simulink model "eCS_Algo_Simulation_2015b_opti - original"  (R2015b)
settings: Solver=ode1  StartTime=0.0  StopTime=3  FixedStep=1/80000  RelTol=1e-3
PreLoadFcn:
  | if exist('tl_preloadfcn','file'), tl_preloadfcn(gcs,402); end
PostLoadFcn:
  | , if any(exist('dsrtsu_mdlpostloadfcn', 'file') == [2, 3, 6]), try dsrtsu_mdlpostloadfcn('Execute', bdroot); catch fprintf('Error in PostLoadFcn (dsrtsu_mdlpostloadfcn) for model "%s":\n %s\n', bdroot, lasterr); end, end,
  | if exist('tl_postloadfcn','file'), tl_postloadfcn(gcs,402); end
InitFcn:
  | Omegan=1.3024e+03;
  | xi=0.9; %0.48
  | K=0.1931;
  | K1=0.0198;
  | TauLocked=0.00255;
  | TauUnLocked=0.0042;
  | Kp=1/(2*K1);
  | Ki=Kp/((TauLocked+TauUnLocked)/2);
  | if exist('tlds_init','file'), tlds_init(gcs); end
StartFcn:
  | if exist('tlds_start','file'), tlds_start(gcs); end
StopFcn:
  | if exist('tlds_stop','file'), tlds_stop(gcs); end
model workspace (MAT data in the model file):
  au8PrevExecProfile = [0 0 0 0 0 0]
values from neighbouring files (symbols this model uses):
  AccSensor = 5    [Parameter_eCS_Algo.m]
  AlgoType = 0    [Parameter_eCS_Algo.m]
  Cxy = 1*0.017    (= 0.017)    [Acc_Init_SelV1.m]
  Cxz = 1*0.017    (= 0.017)    [Acc_Init_SelV1.m]
  Cyx = 1*0.017    (= 0.017)    [Acc_Init_SelV1.m]
  Cyz = 1*0.017    (= 0.017)    [Acc_Init_SelV1.m]
  Czx = 1*0.017    (= 0.017)    [Acc_Init_SelV1.m]
  Czy = 1*0.017    (= 0.017)    [Acc_Init_SelV1.m]
  Forced_Oscillation = 0    [Parameter_eCS_Algo.m]    (also in run_Rotation_sim.m = run)
  FreqTemperature = 10    [Acc_Init_SelV1.m]
  MaxSensorOffset = 0.3    [Acc_Init_SelV1.m]
  Mean_x_noise = 4e-3    (= 0.004)    [Acc_Init_SelV1.m]
  Mean_y_noise = 4e-3    (= 0.004)    [Acc_Init_SelV1.m]
  Mean_z_noise = 4e-3    (= 0.004)    [Acc_Init_SelV1.m]
  ODR = 8000    [Acc_Init_SelV1.m]
  offsetcorrection_on_off = 0    [Parameter_eCS_Algo.m]
  phi_pulse_rotation = 0    [Parameter_eCS_Algo.m]    (also in run_Rotation_sim.m = angle)
  pulsetype = 2    [Parameter_eCS_Algo.m]    (also in run_simulation.m = j; run_simulation_ActiveX.m = j)
  Range = 4    [Acc_Init_SelV1.m]
  sensitivity_optimisation = 0    [Parameter_eCS_Algo.m]
  TempBias = 0    [Acc_Init_SelV1.m]
  TemperatureAmp = 0    [Acc_Init_SelV1.m]
  Var_x_noise = 1.84e-9    (= 1.84e-09)    [Acc_Init_SelV1.m]
  Var_y_noise = 2.025e-09    [Acc_Init_SelV1.m]
  Var_z_noise = 1.374e-09    [Acc_Init_SelV1.m]
  w_x = 2*pi*F_x    (= 376.991118431)    [Acc_Init_SelV1.m]
  w_y = 2*pi*F_y    (= 376.991118431)    [Acc_Init_SelV1.m]
  w_z = 2*pi*F_z    (= 376.991118431)    [Acc_Init_SelV1.m]
  x_max_temp_drift = 0.061    [Acc_Init_SelV1.m]
  x_offset_enable = 0    [Acc_Init_SelV1.m]
  x_run_to_run_drift = 0.0    (= 0)    [Acc_Init_SelV1.m]
  x_temp_co_drift = 0.000    (= 0)    [Acc_Init_SelV1.m]
  Xi_x = 0.7    [Acc_Init_SelV1.m]
  Xi_y = 0.7    [Acc_Init_SelV1.m]
  Xi_z = 0.7    [Acc_Init_SelV1.m]
  y_max_temp_drift = 0.061    [Acc_Init_SelV1.m]
  y_offset_enable = 0    [Acc_Init_SelV1.m]
  y_run_to_run_drift = 0.0    (= 0)    [Acc_Init_SelV1.m]
  y_temp_co_drift = 0.000    (= 0)    [Acc_Init_SelV1.m]
  z_max_temp_drift = 0.13    [Acc_Init_SelV1.m]
  z_offset_enable = 0    [Acc_Init_SelV1.m]
  z_run_to_run_drift = 0.0    (= 0)    [Acc_Init_SelV1.m]
  z_temp_co_drift = 0.000    (= 0)    [Acc_Init_SelV1.m]
undefined symbols (not defined in the file or in its folder): ddv, DiscIntNeverNeededParam, gmw_roada_x__m_s__, gmw_roada_y__m_s__, gmw_roadtime_2kHz, KSF_50_a_x, KSF_50_a_y, KSF_50_time, KSG_30_a_x, KSG_30_a_y, KSG_30_time, Meldorf_HindenburgstraAcceleration_x__m_s_2_, Meldorf_HindenburgstraAcceleration_y__m_s_2_, Meldorf_HindenburgstraAcceleration_z__m_s_2_, Meldorf_HindenburgstraTime__s_, pulse_FF27, pulse_MPDB, pulse_ODB40, pulse_ODB64, pulse_USNCAP, pulsetime_FF27, pulsetime_MPDB, pulsetime_ODB40, pulsetime_ODB64, pulsetime_USNCAP, Rauasphalt_60_a_x, Rauasphalt_60_a_y, Rauasphalt_60_time, sigbuilder_block, VW_416_2kHza_x_2kHz, VW_416_2kHza_y_2kHz, VW_416_2kHztime_2kHz
libraries: simulink x20, tllib x16, tl_autosar_lib x12, simulink_extras x7, LIB_TF_G_12_StepControl x2, LIB_TF_G_111 x1, LIB_TF_G_112 x1
(part 9 of 9)

== system eCS_Algo_Simulation_2015b_opti - original/SAD/Subsystem/SAD/SAD/SAD_runMainFunction/SAD mainfunction/ComputeDutyCycle/UnlockRequest/scp_GetCurrent ==
  u8TypeOfMeasure : Inport  PortDimensions=1  mask(TL_Inport){data={'autosar',{'useautosarcommunication',1,'kind',5,'operationargument','AUTOLIV/AdcIf_DataDictionnary/ClientServerInterfaces/icsConvertedAdcService/Operations/getMeasure/OperationArguments/u8TypeOfMeasure'},'date',738771.48216400458}}
      settings: CopyFcn=if exist('tl_reset_reviewflag') == 2, tl_reset_reviewflag(gcbh); end  DeleteFcn=if exist('delete_tlblock','file')==2,delete_tlblock(gcbh);end  NameChangeFcn=if exist('rename_tlblock','file')==2,rename_tlblock(gcbh);end  OpenFcn=if exist('tl_open_blockdlg','file')==2,tl_open_blockdlg(gcbh);else,open_system(gcbh,'parameter');end
      mask Help: eval(['if exist(''tl_online_help'',''file'') == 2, tl_online_help(''Topic'',''TL_Inport''),else, web([''jar:file:///'',matlabroot,''/help/toolbox/simulink/help.jar!/slref/' lower(get_param(gcbh,'Blocktype')) '.html''], ''-helpbrowser''),end'])
      mask Display: plot([0.2 0.35 NaN 0.65 0.8],[0 1 NaN 0 1]);
  Data Store Read : DataStoreRead  mask(TL_DataStoreRead){data={'date',738672.58044925926}}
      settings: DeleteFcn=if exist('delete_tlblock','file')==2,delete_tlblock(gcbh);end  NameChangeFcn=if exist('rename_tlblock','file')==2,rename_tlblock(gcbh);end  OpenFcn=if exist('tl_open_blockdlg','file')==2,tl_open_blockdlg(gcbh);else,open_system(gcbh,'parameter');end
      mask Help: eval(['if exist(''tl_online_help'',''file'') == 2, tl_online_help(''Topic'',''TL_DataStoreRead''),else, web([''jar:file:///'',matlabroot,''/help/toolbox/simulink/help.jar!/slref/' lower(get_param(gcbh,'Blocktype')) '.html''], ''-helpbrowser''),end'])
      mask Display: plot([-0.1, 1.05, NaN, -0.1, 1.05],[.01, .01, NaN, .99, .99]);
  Selector : Selector  IndexMode=Zero-based  InputPortWidth=6  IndexOptions=Index vector (port)  Indices=[1 3]  OutputSizes=1
  ServerCallPoint : tllib/Function  data={'autosar',{'useautosarspecification',1,'functionrole',3,'clientport','pclSolenoidCurrent','operation','getMeasure','clientsoftwarecomponent','AUTOLIV/SoftwareComponents/SAD/SAD'},'date',738770.65144107642}  displayString=|
      | OPERATION CALL
      | (SYNCHRONOUS)
  u16Current : Outport  PortDimensions=1  mask(TL_Outport){data={'autosar',{'useautosarcommunication',1,'kind',5,'operationargument','AUTOLIV/AdcIf_DataDictionnary/ClientServerInterfaces/icsConvertedAdcService/Operations/getMeasure/OperationArguments/u16Measure'},'date',738771.47910792823}}
      settings: CopyFcn=if exist('tl_reset_reviewflag') == 2, tl_reset_reviewflag(gcbh); end  DeleteFcn=if exist('delete_tlblock','file')==2,delete_tlblock(gcbh);end  NameChangeFcn=if exist('rename_tlblock','file')==2,rename_tlblock(gcbh);end  OpenFcn=if exist('tl_open_blockdlg','file')==2,tl_open_blockdlg(gcbh);else,open_system(gcbh,'parameter');end
      mask Help: eval(['if exist(''tl_online_help'',''file'') == 2, tl_online_help(''Topic'',''TL_Outport''),else, web([''jar:file:///'',matlabroot,''/help/toolbox/simulink/help.jar!/slref/' lower(get_param(gcbh,'Blocktype')) '.html''], ''-helpbrowser''),end'])
      mask Display: plot([0.2 0.35 NaN 0.65 0.8],[0 1 NaN 0 1]);
  wires:
  Selector/1 -> u16Current/1
  Data Store Read/1 -> Selector/1
  u8TypeOfMeasure/1 -> Selector/2

== system eCS_Algo_Simulation_2015b_opti - original/eCS/Subsystem/eCS/eCS/eCS_runMainFunction/Crash Acceleration/Acceleration Clipping/If Action Subsystem/Clear Trigger  ==
  u16OldTimer : Inport
  Action Port : ActionPort  ActionType=then
  Constant1 : Constant  Value=0  mask(TL_Constant){data={'date',738573.7192003472}}
      settings: CopyFcn=if exist('tl_reset_reviewflag') == 2, tl_reset_reviewflag(gcbh); end  DeleteFcn=if exist('delete_tlblock','file')==2,delete_tlblock(gcbh);end  NameChangeFcn=if exist('rename_tlblock','file')==2,rename_tlblock(gcbh);end  OpenFcn=if exist('tl_open_blockdlg','file')==2,tl_open_blockdlg(gcbh);else,open_system(gcbh,'parameter');end
      mask Help: eval(['if exist(''tl_online_help'',''file'') == 2, tl_online_help(''Topic'',''TL_Constant''),else, web([''jar:file:///'',matlabroot,''/help/toolbox/simulink/help.jar!/slref/' lower(get_param(gcbh,'Blocktype')) '.html''], ''-helpbrowser''),end'])
      mask Display: plot([-0.1, 1.05, NaN, -0.1, 1.05],[.01, .01, NaN, .99, .99]);
  Trigger : Outport  InitialOutput=0
  u16Timer : Outport  Port=2  InitialOutput=0
  wires:
  Constant1/1 -> Trigger/1
  u16OldTimer/1 -> u16Timer/1

== system eCS_Algo_Simulation_2015b_opti - original/eCS/Subsystem/eCS/eCS/eCS_runMainFunction/Crash Acceleration/Acceleration Clipping/If Action Subsystem/Decrease Timer ==
  u16OldTimer : Inport
  u8OldTrigger : Inport  Port=2
  Action Port : ActionPort  ActionType=else
  Constant : Constant  mask(TL_Constant){data={'date',738573.71920056711}}
      settings: CopyFcn=if exist('tl_reset_reviewflag') == 2, tl_reset_reviewflag(gcbh); end  DeleteFcn=if exist('delete_tlblock','file')==2,delete_tlblock(gcbh);end  NameChangeFcn=if exist('rename_tlblock','file')==2,rename_tlblock(gcbh);end  OpenFcn=if exist('tl_open_blockdlg','file')==2,tl_open_blockdlg(gcbh);else,open_system(gcbh,'parameter');end
      mask Help: eval(['if exist(''tl_online_help'',''file'') == 2, tl_online_help(''Topic'',''TL_Constant''),else, web([''jar:file:///'',matlabroot,''/help/toolbox/simulink/help.jar!/slref/' lower(get_param(gcbh,'Blocktype')) '.html''], ''-helpbrowser''),end'])
      mask Display: plot([-0.1, 1.05, NaN, -0.1, 1.05],[.01, .01, NaN, .99, .99]);
  Constant1 : Constant  Value=0  mask(TL_Constant){data={'date',738573.71920068283}}
      settings: CopyFcn=if exist('tl_reset_reviewflag') == 2, tl_reset_reviewflag(gcbh); end  DeleteFcn=if exist('delete_tlblock','file')==2,delete_tlblock(gcbh);end  NameChangeFcn=if exist('rename_tlblock','file')==2,rename_tlblock(gcbh);end  OpenFcn=if exist('tl_open_blockdlg','file')==2,tl_open_blockdlg(gcbh);else,open_system(gcbh,'parameter');end
      mask Help: eval(['if exist(''tl_online_help'',''file'') == 2, tl_online_help(''Topic'',''TL_Constant''),else, web([''jar:file:///'',matlabroot,''/help/toolbox/simulink/help.jar!/slref/' lower(get_param(gcbh,'Blocktype')) '.html''], ''-helpbrowser''),end'])
      mask Display: plot([-0.1, 1.05, NaN, -0.1, 1.05],[.01, .01, NaN, .99, .99]);
  HoldingTimer : Switch  Criteria=u2 ~= 0  mask(TL_Switch){data={'output',{'type','UInt16'},'date',738573.71920091438}}
      settings: CopyFcn=if exist('tl_reset_reviewflag') == 2, tl_reset_reviewflag(gcbh); end  DeleteFcn=if exist('delete_tlblock','file')==2,delete_tlblock(gcbh);end  NameChangeFcn=if exist('rename_tlblock','file')==2,rename_tlblock(gcbh);end  OpenFcn=if exist('tl_open_blockdlg','file')==2,tl_open_blockdlg(gcbh);else,open_system(gcbh,'parameter');end
      mask Help: eval(['if exist(''tl_online_help'',''file'') == 2, tl_online_help(''Topic'',''TL_Switch''),else, web([''jar:file:///'',matlabroot,''/help/toolbox/simulink/help.jar!/slref/' lower(get_param(gcbh,'Blocktype')) '.html''], ''-helpbrowser''),end'])
      mask Display: plot([-0.1, 1.05, NaN, -0.1, 1.05],[.01, .01, NaN, .99, .99]);
  Sum : Sum  Inputs=+-  mask(TL_Sum){data={'output',{'type','UInt16'},'date',738573.71920103009}}
      settings: CopyFcn=if exist('tl_reset_reviewflag') == 2, tl_reset_reviewflag(gcbh); end  DeleteFcn=if exist('delete_tlblock','file')==2,delete_tlblock(gcbh);end  NameChangeFcn=if exist('rename_tlblock','file')==2,rename_tlblock(gcbh);end  OpenFcn=if exist('tl_open_blockdlg','file')==2,tl_open_blockdlg(gcbh);else,open_system(gcbh,'parameter');end
      mask Help: eval(['if exist(''tl_online_help'',''file'') == 2, tl_online_help(''Topic'',''TL_Sum''),else, web([''jar:file:///'',matlabroot,''/help/toolbox/simulink/help.jar!/slref/' lower(get_param(gcbh,'Blocktype')) '.html''], ''-helpbrowser''),end'])
      mask Display: plot([-0.1, 1.05, NaN, -0.1, 1.05],[.01, .01, NaN, .99, .99]);
  u16Timer : Outport  InitialOutput=0
  Trigger : Outport  Port=2  InitialOutput=0
  wires:
  u16OldTimer/1 -> Sum/1, HoldingTimer/2
  HoldingTimer/1 -> u16Timer/1
  Constant/1 -> Sum/2
  Sum/1 -> HoldingTimer/1
  Constant1/1 -> HoldingTimer/3
  u8OldTrigger/1 -> Trigger/1

== matlab function eCS_Algo_Simulation_2015b_opti - original/retractor locking trigger ==
  settings: updateMethod=DISCRETE
  data: trigger_solenoid input; s input; s_mech_locking input; trigger_retractor output; time input; triggertime_retractor output; s_locking output
function [trigger_retractor,triggertime_retractor,s_locking]     = retractor_locking_trigger(trigger_solenoid, s, s_mech_locking,time)

%local variable declaration
persistent s_store
persistent trigger_old
persistent trigger_intern
persistent t_store
persistent s_locking_intern
persistent once

% Initialisation
if isempty(s_store)
    s_store=10000;
    trigger_old=0;
    trigger_intern=0;    
    t_store=0;
    s_locking_intern=0;
    once=0;
end


%main
if and(trigger_old==0, trigger_solenoid==1)
    trigger_old=1;
    s_store=s;
    %s_locking_intern=s;
end

if and(s-s_store>s_mech_locking , once==0)
    once=1;
    trigger_intern=1;
    t_store=time;
    s_locking_intern=s;
end

% Output 
trigger_retractor=trigger_intern;
triggertime_retractor=t_store * 1000;
s_locking=s_locking_intern;

== matlab function eCS_Algo_Simulation_2015b_opti - original/trigger travels, times and counts ==
  settings: updateMethod=DISCRETE
  data: s_locking output; trigger input; s input; triggertime output; time input; triggercounts output; triggerCountsTL output; eCSTrigger input; triggerTimeTL output
function [s_locking , triggertime, triggercounts, triggerCountsTL, triggerTimeTL]     = triggertime(trigger , s , time, eCSTrigger)
%Input a trigger signal (0 to 1)n and calculate/output the triggertime in ms
%local variable declaration
persistent trigger_once
persistent trigger_once_TL
persistent triggertime_intern
persistent triggertime_intern_TL
persistent s_locking_intern
persistent triggercounts_intern
persistent trigger_old
persistent triggercounts_intern_tl
persistent prevTrigger

% Initialisation
if isempty(trigger_once)
   trigger_once=0;
   trigger_once_TL = 0;
   triggertime_intern = 0 ;
   triggertime_intern_TL = 0;
   s_locking_intern = 0 ;   
   triggercounts_intern = 0 ;
   trigger_old=0; 
   triggercounts_intern_tl = 0;
   prevTrigger = 0;
end


%main

    %one-time detection of first trigger to set triggertime and travel
    if and (trigger_once==0 , trigger==1)
        trigger_once=1;
        triggertime_intern=time*1000;
        s_locking_intern = s ;  
    end
    
    %one-time detection of first trigger to set triggertime and travel
    if and (trigger_once_TL==0 , eCSTrigger==1)
        trigger_once_TL=1;
        triggertime_intern_TL=time*1000; 
    end

    %count the number of triggers
    if trigger_old~=trigger
        trigger_old=trigger;
        triggercounts_intern=triggercounts_intern+0.5;
    end
    
    if prevTrigger~=eCSTrigger
        prevTrigger = eCSTrigger;
        triggercounts_intern_tl = triggercounts_intern_tl + 0.5;
    end
    
    
% Output 
triggertime=triggertime_intern;
s_locking=s_locking_intern;
triggercounts=triggercounts_intern;
triggerCountsTL = triggercounts_intern_tl;
triggerTimeTL = triggertime_intern_TL;

== matlab function eCS_Algo_Simulation_2015b_opti - original/trigger travels, times and counts1 ==
  settings: updateMethod=DISCRETE
  data: s_locking output; trigger input; s input; triggertime output; time input; triggercounts output
function [s_locking , triggertime, triggercounts]     = triggertime(trigger , s , time)
%Input a trigger signal (0 to 1)n and calculate/output the triggertime in ms
%local variable declaration
persistent trigger_once
persistent triggertime_intern
persistent s_locking_intern
persistent triggercounts_intern
persistent trigger_old

% Initialisation
if isempty(trigger_once)
   trigger_once=0;
   triggertime_intern = 0 ;
   s_locking_intern = 0 ;   
   triggercounts_intern = 0 ;
   trigger_old=0;   
end


%main

    %one-time detection of first trigger to set triggertime and travel
    if and (trigger_once==0 , trigger==1)
        trigger_once=1;
        triggertime_intern=time*1000;
        s_locking_intern = s ;  
    end

    %count the number of triggers
    if trigger_old~=trigger
        trigger_old=trigger;
        triggercounts_intern=triggercounts_intern+0.5;
    end    
    
    
% Output 
triggertime=triggertime_intern;
s_locking=s_locking_intern;
triggercounts=triggercounts_intern;

== matlab function eCS_Algo_Simulation_2015b_opti - original/eCS Algo new2/Trigger_hold_time ==
  data: trigger_in input; trigger_out output; time input; time_delay input; delta_t_min_since_previous_unlock input; time_delay_out output; a_z_axis input; counter_out output; timeSinceLastUnlock output
function [trigger_out,time_delay_out, counter_out, timeSinceLastUnlock]    = Trigger_hold_time(trigger_in,time,time_delay,delta_t_min_since_previous_unlock,a_z_axis)
%no impact on trigger change from 0 to 1 (-->locking)
%delays the time for the trigger signal from 1 to 0 (-->unlocking) to avoid
%too many subsequent locking in a certain time

%local variable declaration
persistent time_store
persistent trigger_intern
persistent time_delay_intern
persistent time_since_last_unlock

% Initialisation
if isempty(time_store)
   time_store = 0 ;
   trigger_intern = 0 ;
   time_delay_intern = time_delay ;
   time_since_last_unlock = 10;
end

% main
if trigger_in==1
    time_store=time;
    trigger_intern=trigger_in;
end

if a_z_axis>=-0.5       %Rolllover-check: if Z-axis >0.5g then reset unlocking timer
    time_store=time;
end    

if trigger_intern==0
    time_since_last_unlock = time-time_store;
end


if time_since_last_unlock<((delta_t_min_since_previous_unlock)/1000)
   time_delay_intern = time_delay+1000 ;     %additional delay 1000ms when next locking happens too fast
else    
   time_delay_intern = time_delay;    
end

if time>=(time_store+ (time_delay_intern/1000) )
    trigger_intern=trigger_in;
end

% Output
trigger_out=trigger_intern;
time_delay_out=time_delay_intern;
counter_out = (time_store+ (time_delay_intern/1000)) - time;
timeSinceLastUnlock = time_since_last_unlock;

== matlab function eCS_Algo_Simulation_2015b_opti - original/eCS Algo new2/aceleration clipping trigger ==
  settings: updateMethod=DISCRETE
  data: trigger_out output; pulse_in input; triggertime output; time input; no_of_samples input; a_threshold input
function [trigger_out , triggertime]     = acceleration_clipping_trigger(pulse_in, time, no_of_samples, a_threshold)
%Inputthe pulse signal and count the number of subsequent samples above the
%acceleration threshold - when the numer of allowed samples are reached,
%then the trigger_out goes from 1 to 0 for a certain hold-time
%intention is to detect a crahs-pulse a.s.a.p when the acceleration signal
%excceeds a certain threshold

%local variable declaration
persistent trigger_intern
persistent triggertime_intern
persistent samples_counter


% Initialisation
if isempty(trigger_intern)
   trigger_intern=0;
   triggertime_intern = 0 ;
   samples_counter = 0 ;   
end


%main
if pulse_in>=a_threshold
    samples_counter = samples_counter+1 ;
else
    samples_counter=0;
end



if  and( samples_counter>=no_of_samples , trigger_intern==0)
    trigger_intern=1;
    triggertime_intern=time*1000;
end

if and ( and( samples_counter<no_of_samples , trigger_intern==1) , (time-(triggertime_intern/1000)) > 0.1 )
    trigger_intern=0;
end
% Output
trigger_out=trigger_intern;
triggertime=triggertime_intern;

== matlab function eCS_Algo_Simulation_2015b_opti - original/solenoid time delay ==
  settings: updateMethod=DISCRETE
  data: trigger input; trigger_out output; time input; dt_to_lock input; dt_to_unlock input
function trigger_out     = solenoid_time_delay(trigger,time,dt_to_lock,dt_to_unlock)

%local variable declaration
persistent trigger_old
persistent trigger_intern
persistent t_on
persistent t_off


% Initialisation
if isempty(trigger_old)
   trigger_old=0;
   trigger_intern = 0 ;   
   t_on=-1;      %delay time for switching on
   t_off=-1;      %delay time for switching off   
end


%main
if and (trigger_old==0 , trigger==1)
    trigger_old=1;
    t_on=time;
    t_off=-1;
end
if and (trigger_old==1 , trigger==0)
    trigger_old=0;
    t_off=time;
    t_on=-1;    
end

if and ( time-t_on>=dt_to_lock/1000 , time-t_on<1)
       trigger_intern=1; 
end    
if and ( time-t_off>=dt_to_unlock/1000 , time-t_off<1)
       trigger_intern=0; 
end   

% Output 
trigger_out=trigger_intern;
